simulink model "simulink_model_assignment1"  (R2022b)
settings: Solver=VariableStepAuto  StartTime=0.0  StopTime=1  RelTol=1e-3
values from neighbouring files (symbols this model uses):
  beta = 1.19 * 10^(-7)    (= 1.19e-07)    [parameters.m]
  J = 3.88*10^(-5)    (= 3.88e-05)    [parameters.m]
  k = 0.051    [parameters.m]
  L = 3.39*10^(-3)    (= 0.00339)    [parameters.m]
  Rc_Rr = 1.15    [parameters.m]
settings Model: Creator=rappl  LastModifiedBy=Javier
settings ModelReferenceCC: EnableRefExpFcnMdlSchedulingChecks=on

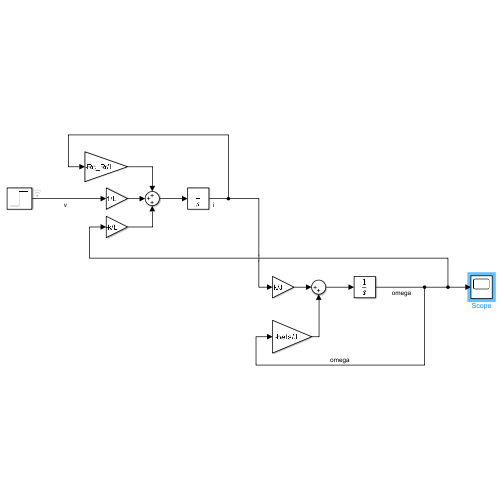
[thumbnail: Simulink's stored preview of the top-level diagram]
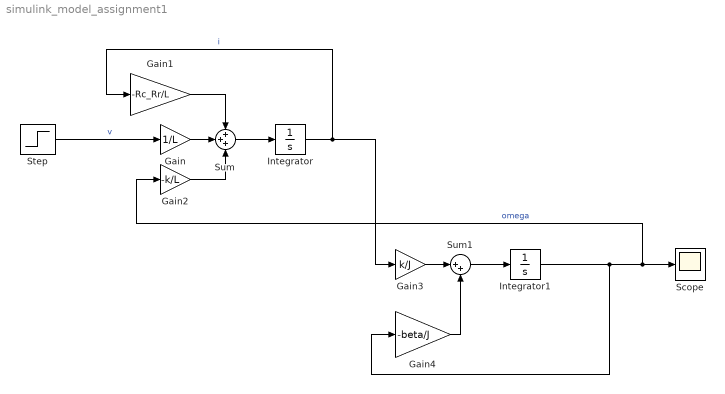
== system simulink_model_assignment1 ==
  Gain : Gain  Gain=1/L
  Gain1 : Gain  Gain=-Rc_Rr/L
  Gain2 : Gain  Gain=-k/L
  Gain3 : Gain  Gain=k/J
  Gain4 : Gain  Gain=-beta/J
  Integrator : Integrator
  Integrator1 : Integrator
  Scope : Scope
  Step : Step  Time=0  SampleTime=0
  Sum : Sum  Inputs=+++
  Sum1 : Sum  Inputs=|++
  wires:
  Sum/1 -> Integrator/1
  Sum1/1 -> Integrator1/1
  Integrator1/1 -> Scope/1, Gain2/1, Gain4/1  "omega"
  Gain/1 -> Sum/2
  Gain2/1 -> Sum/3
  Gain1/1 -> Sum/1
  Integrator/1 -> Gain3/1, Gain1/1  "i"
  Step/1 -> Gain/1  "v"
  Gain3/1 -> Sum1/1
  Gain4/1 -> Sum1/2
